simulink model "skewSine"  (R2018a)
settings: Solver=FixedStepAuto  StartTime=0.0  StopTime=t_end  FixedStep=ts  RelTol=1e-3
values from neighbouring files (symbols this model uses):
  ampl = 10    [Tflex_PID_init.m]
  seed = 35    [Tflex_PID_init.m]
  sp_ts = 2.5    [Tflex_PID_init.m]
  tm = 2    [Tflex_PID_init.m]
settings Model: Creator=wout7  LastModifiedBy=wout7
settings DebuggingCC: LibraryContextMissingDiagnostic=warning
settings SFSimCC: SimUseLocalCustomCode=on
settings RTWCC: RTWUseLocalCustomCode=on

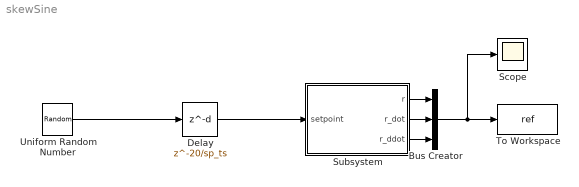
== system skewSine ==
  Bus Creator : BusCreator  Inputs=3
  Delay : Delay  DelayLength=20/sp_ts  SampleTime=sp_ts
  Scope : Scope
  Subsystem : Subsystem
  To Workspace : ToWorkspace  VariableName=ref  SaveFormat=Timeseries  SampleTime=-1
  Uniform Random Number : UniformRandomNumber  Minimum=-ampl  Maximum=ampl  Seed=seed  SampleTime=sp_ts
  wires:
  Subsystem/1(r) -> Bus Creator/1
  Subsystem/2(r_dot) -> Bus Creator/2
  Subsystem/3(r_ddot) -> Bus Creator/3
  Bus Creator/1 -> To Workspace/1, Scope/1
  Uniform Random Number/1 -> Delay/1
  Delay/1 -> Subsystem/1(setpoint)

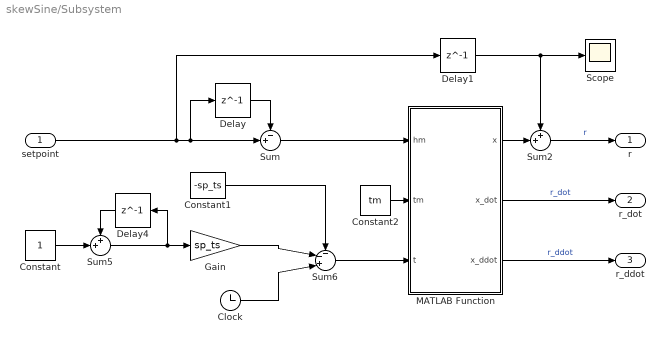
== system skewSine/Subsystem ==
  setpoint : Inport
  Clock : Clock
  Constant : Constant  SampleTime=sp_ts
  Constant1 : Constant  Value=-sp_ts  SampleTime=sp_ts
  Constant2 : Constant  Value=tm  SampleTime=sp_ts
  Delay : Delay  DelayLength=1  InitialCondition=0  SampleTime=sp_ts
  Delay1 : Delay  DelayLength=1  InitialCondition=0  SampleTime=sp_ts
  Delay4 : Delay  DelayLength=1  InitialCondition=0  SampleTime=sp_ts
  Gain : Gain  Gain=sp_ts
  MATLAB Function : MATLAB Function  TreatAsAtomicUnit=on
  Scope : Scope
  Sum : Sum  Inputs=-+|
  Sum2 : Sum  Inputs=++|
  Sum5 : Sum  Inputs=++|
  Sum6 : Sum  Inputs=--+|
  r : Outport
  r_dot : Outport  Port=2
  r_ddot : Outport  Port=3
  wires:
  Constant2/1 -> MATLAB Function/2(tm)
  MATLAB Function/1(x) -> Sum2/2
  Delay1/1 -> Scope/1, Sum2/1
  Delay4/1 -> Sum5/1
  Sum/1 -> MATLAB Function/1(hm)
  setpoint/1 -> Delay1/1, Delay/1, Sum/2
  Sum2/1 -> r/1  "r"
  Sum5/1 -> Delay4/1, Gain/1
  Constant/1 -> Sum5/2
  MATLAB Function/3(x_ddot) -> r_ddot/1  "r_ddot"
  Clock/1 -> Sum6/3
  Sum6/1 -> MATLAB Function/3(t)
  Delay/1 -> Sum/1
  Gain/1 -> Sum6/2
  Constant1/1 -> Sum6/1
  MATLAB Function/2(x_dot) -> r_dot/1  "r_dot"

== matlab function skewSine/Subsystem/MATLAB Function ==
  settings: updateMethod=DISCRETE  sampleTime=ts
  data: hm input; x output; tm input; t input; x_dot output; x_ddot output
function [x,x_dot,x_ddot] = skewSine(hm,tm,t)

if (t>=0) && (t<=tm)
    x      = hm/tm*t - hm/(2*pi)*sin(2*pi/tm*t);
    x_dot  = hm/tm - hm/tm*cos(2*pi/tm*t);
    x_ddot = 2*pi*hm/(tm^2)*sin(2*pi/tm*t);
else
    x      = hm;
    x_dot  = 0;
    x_ddot = 0;
end
